simulink model "comfortController"  (R2015b)
settings: Solver=VariableStepAuto  StartTime=0.0  StopTime=inf  RelTol=1e-3
model workspace: external: MAT-File /home/sprinkle/ros15/trunk/gazebo_workspace/src/azcar_sim/simulink/lod.mat (data not in the file)
libraries: robotlib x2, simulink x1
settings Model: Creator=sprinkle  LastModifiedBy=sprinkle

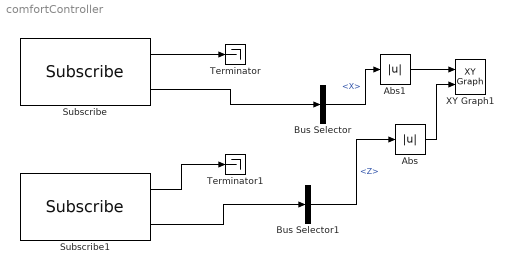
== system comfortController ==
  Abs : Abs
  Abs1 : Abs
  Bus Selector : BusSelector  OutputSignals=Linear.X
  Bus Selector1 : BusSelector  OutputSignals=Torque.Z
  Subscribe : robotlib/Subscribe  SourceLibraryInfo=This block requires Robotics System Toolbox  topicSource=Select from ROS network  topic=/azcar_sim/vel  messageType=geometry_msgs/Twist  sampleTime=-1  messageQueueLength=1
  Subscribe1 : robotlib/Subscribe  SourceLibraryInfo=This block requires Robotics System Toolbox  topicSource=Select from ROS network  topic=/azcar_sim/steering  messageType=geometry_msgs/Wrench  sampleTime=-1  messageQueueLength=1
  Terminator : Terminator
  Terminator1 : Terminator
  XY Graph1 : simulink/Sinks/XY Graph  xmin=-1  xmax=30  ymin=-0.1  ymax=0.4  st=-1
  wires:
  Subscribe/2 -> Bus Selector/1
  Subscribe1/2 -> Bus Selector1/1
  Subscribe/1 -> Terminator/1
  Subscribe1/1 -> Terminator1/1
  Bus Selector/1 -> Abs1/1  "<X>"
  Bus Selector1/1 -> Abs/1  "<Z>"
  Abs/1 -> XY Graph1/2
  Abs1/1 -> XY Graph1/1
